simulink model "bh_2dof_NP_CONTROLLED_compare_lagr_sm"  (R2017a)
settings: Solver=ode45  StartTime=0.0  StopTime=70  FixedStep=0.001  RelTol=1e-7  EnableMultiTasking=on
values from neighbouring files (symbols this model uses):
  theta1_0 = 0    [bh_SIMPARAMS_for_2dof_NP_Control_sim.m]
  theta1_dot_0 = 0    [bh_SIMPARAMS_for_2dof_NP_Control_sim.m]
  theta4_0 = 0    [bh_SIMPARAMS_for_2dof_NP_Control_sim.m]
  theta4_dot_0 = 0    [bh_SIMPARAMS_for_2dof_NP_Control_sim.m]
undefined symbols (not defined in the file or in its folder): b1_damp, b4_damp, g, Hz, L1x, L1y, L1z, mass1, mass4, Rturn, sigbuilder_block, X, Y, Z
libraries: simulink_extras x30, sm_lib x13, nesl_utility x9, simulink x8, discretizing x2
(part 2 of 2)

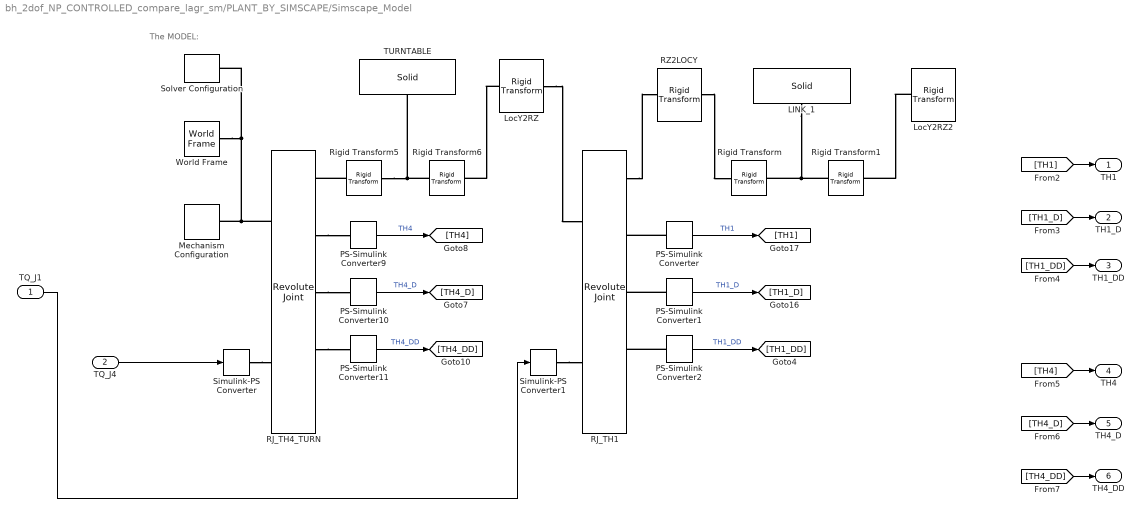
== system bh_2dof_NP_CONTROLLED_compare_lagr_sm/PLANT_BY_SIMSCAPE/Simscape_Model ==
  note: The MODEL:
  "TQ_J1 " : Inport
  TQ_J4 : Inport  Port=2
  LINK_1 : sm_lib/Body Elements/Solid  InertiaType=CalculateFromGeometry  Mass=1  MassUnits=kg  CenterOfMass=[0 0 0]  CenterOfMassUnits=m  MomentsOfInertia=[1 1 1]  MomentsOfInertiaUnits=kg*m^2  ProductsOfInertia=[0 0 0]  ProductsOfInertiaUnits=kg*m^2  DensityBased=on  Density=density  DensityUnits=kg/(m^3)  DoExposeReferenceFrame=on  SerializedFrames=<Frames/>  GraphicType=FromGeometry  MarkerShape=Sphere  MarkerSize=10  GraphicVisPropType=SimpleVisualProperties  GraphicDiffuseColor=[0.2 0.2 1.0]  GraphicSpecularColor=[0.5 0.5 0.5 1.0]  GraphicAmbientColor=[0.15 0.15 0.15 1.0]  GraphicEmissiveColor=[0.0 0.0 0.0 1.0]  GraphicShininess=75  GraphicOpacity=1.0  GeometryShape=Brick  RectangleSize=[1 1]  RectangleSizeUnits=m  BrickDimensions=[L1x, L1y, L1z ]  BrickDimensionUnits=m  CylinderRadius=1  CylinderRadiusUnits=m  CylinderLength=1  CylinderLengthUnits=m  SphereRadius=1  SphereRadiusUnits=m  EllipsoidRadii=[1 1 1]  EllipsoidRadiiUnits=m  ExtrusionCrossSection=[1 1; -1 1; -1 -1; 1 -1]  ExtrusionCrossSectionUnits=m  ExtrusionLength=1  ExtrusionLengthUnits=m  PolygonNumSides=3  PolygonOuterRadius=1  PolygonOuterRadiusUnits=m  ExtGeomFileType=STEP  ExtGeomFileUnits=m  RevolutionCrossSection=[1 1; 1 -1; 2 -1; 2 1]  RevolutionCrossSectionUnits=m  RevolutionExtent=Full  RevolutionAngle=180  RevolutionAngleUnits=deg
  LocY2RZ : sm_lib/Frames and Transforms/Rigid Transform  TranslationMethod=None  TranslationStandardOffset=Hz/2  TranslationLengthUnit=m  TranslationStandardAxis=+Z  TranslationCartesianOffset=[0 0 0]  TranslationROffset=0  TranslationROffsetUnits=m  TranslationZOffset=0  TranslationZOffsetUnits=m  TranslationThetaOffset=0  TranslationThetaOffsetUnits=deg  RotationMethod=AlignedAxes  RotationAngleUnits=deg  RotationStandardAxis=+Z  RotationAngle=0.0  RotationArbitraryAxis=[0 0 1]  FollAlignAxisA=+X  BaseAlignAxisA=+Y  FollAlignAxisB=+Y  BaseAlignAxisB=+Z  RotationSequenceAxes=FollowerAxes  RotationSequence=XYX  RotationSequenceAngles=[0 0 0]  RotationSequenceAnglesUnits=deg  RotationMatrix=[1 0 0; 0 1 0; 0 0 1]
  LocY2RZ2 : sm_lib/Frames and Transforms/Rigid Transform  TranslationMethod=None  TranslationStandardOffset=Hz/2  TranslationLengthUnit=m  TranslationStandardAxis=+Z  TranslationCartesianOffset=[0 0 0]  TranslationROffset=0  TranslationROffsetUnits=m  TranslationZOffset=0  TranslationZOffsetUnits=m  TranslationThetaOffset=0  TranslationThetaOffsetUnits=deg  RotationMethod=AlignedAxes  RotationAngleUnits=deg  RotationStandardAxis=+Z  RotationAngle=0.0  RotationArbitraryAxis=[0 0 1]  FollAlignAxisA=+X  BaseAlignAxisA=+Y  FollAlignAxisB=+Y  BaseAlignAxisB=+Z  RotationSequenceAxes=FollowerAxes  RotationSequence=XYX  RotationSequenceAngles=[0 0 0]  RotationSequenceAnglesUnits=deg  RotationMatrix=[1 0 0; 0 1 0; 0 0 1]
  Mechanism Configuration : sm_lib/Utilities/Mechanism Configuration  UniformGravity=Constant  GravityVector=[0 0 -g ]  GravityUnits=m/s^2  LinearizationDelta=1e-4
  PS-Simulink Converter : nesl_utility/PS-Simulink Converter  PhysicalDomain=network_engine_domain  SubClassName=ps_output  LeftPortType=input  RightPortType=output  PseudoPeriodic=off  Frequencies=[]  Unit=rad  AffineConversion=off
  PS-Simulink Converter1 : nesl_utility/PS-Simulink Converter  PhysicalDomain=network_engine_domain  SubClassName=ps_output  LeftPortType=input  RightPortType=output  PseudoPeriodic=off  Frequencies=[]  Unit=rad/s  AffineConversion=off
  PS-Simulink Converter10 : nesl_utility/PS-Simulink Converter  PhysicalDomain=network_engine_domain  SubClassName=ps_output  LeftPortType=input  RightPortType=output  PseudoPeriodic=off  Frequencies=[]  Unit=rad/s  AffineConversion=off
  PS-Simulink Converter11 : nesl_utility/PS-Simulink Converter  PhysicalDomain=network_engine_domain  SubClassName=ps_output  LeftPortType=input  RightPortType=output  PseudoPeriodic=off  Frequencies=[]  Unit=rad/s^2  AffineConversion=off
  PS-Simulink Converter2 : nesl_utility/PS-Simulink Converter  PhysicalDomain=network_engine_domain  SubClassName=ps_output  LeftPortType=input  RightPortType=output  PseudoPeriodic=off  Frequencies=[]  Unit=rad/s^2  AffineConversion=off
  PS-Simulink Converter9 : nesl_utility/PS-Simulink Converter  PhysicalDomain=network_engine_domain  SubClassName=ps_output  LeftPortType=input  RightPortType=output  PseudoPeriodic=off  Frequencies=[]  Unit=rad  AffineConversion=off
  RJ_TH1 : sm_lib/Joints/Revolute Joint  SenseConstraintForce=on  SenseConstraintForceX=off  SenseConstraintForceY=off  SenseConstraintForceZ=off  SenseConstraintTorque=off  SenseConstraintTorqueX=off  SenseConstraintTorqueY=off  SenseConstraintTorqueZ=off  SenseTotalForce=off  SenseTotalForceX=off  SenseTotalForceY=off  SenseTotalForceZ=off  SenseTotalTorque=off  SenseTotalTorqueX=off  SenseTotalTorqueY=off  SenseTotalTorqueZ=off  CompositeWrenchDir=BaseOnFollower  CompositeWrenchFrame=BaseFrame  EquilibriumPosition=0  EquilibriumPositionUnits=deg  SpringStiffness=0  SpringStiffnessUnits=N*m/deg  DampingCoefficient=b1_damp  DampingCoefficientUnits=N*m/(rad/s)  TorqueActuationMode=InputTorque  MotionActuationMode=ComputedMotion  SensePosition=on  SenseVelocity=on  SenseAcceleration=on  SenseTorqueForce=off  PositionTargetSpecify=on  PositionTargetPriority=Low  PositionTargetValue=theta1_0  PositionTargetValueUnits=rad  VelocityTargetSpecify=on  VelocityTargetPriority=High  VelocityTargetValue=theta1_dot_0  VelocityTargetValueUnits=rad/s
      settings: AttributesFormatString=|
      | %<DampingCoefficient>
      | %<PositionTargetValue>
      | %<VelocityTargetValue>
  RJ_TH4_TURN : sm_lib/Joints/Revolute Joint  SenseConstraintForce=on  SenseConstraintForceX=off  SenseConstraintForceY=off  SenseConstraintForceZ=off  SenseConstraintTorque=off  SenseConstraintTorqueX=off  SenseConstraintTorqueY=off  SenseConstraintTorqueZ=off  SenseTotalForce=off  SenseTotalForceX=off  SenseTotalForceY=off  SenseTotalForceZ=off  SenseTotalTorque=off  SenseTotalTorqueX=off  SenseTotalTorqueY=off  SenseTotalTorqueZ=off  CompositeWrenchDir=BaseOnFollower  CompositeWrenchFrame=BaseFrame  EquilibriumPosition=0  EquilibriumPositionUnits=deg  SpringStiffness=0  SpringStiffnessUnits=N*m/deg  DampingCoefficient=b4_damp  DampingCoefficientUnits=N*m/(rad/s)  TorqueActuationMode=InputTorque  MotionActuationMode=ComputedMotion  SensePosition=on  SenseVelocity=on  SenseAcceleration=on  SenseTorqueForce=off  PositionTargetSpecify=on  PositionTargetPriority=Low  PositionTargetValue=theta4_0  PositionTargetValueUnits=rad  VelocityTargetSpecify=on  VelocityTargetPriority=High  VelocityTargetValue=theta4_dot_0  VelocityTargetValueUnits=rad/s
      settings: AttributesFormatString=|
      | %<DampingCoefficient>
      | %<PositionTargetValue>
      | %<VelocityTargetValue>
  RZ2LOCY : sm_lib/Frames and Transforms/Rigid Transform  TranslationMethod=None  TranslationStandardOffset=Hz/2  TranslationLengthUnit=m  TranslationStandardAxis=+Z  TranslationCartesianOffset=[0 0 0]  TranslationROffset=0  TranslationROffsetUnits=m  TranslationZOffset=0  TranslationZOffsetUnits=m  TranslationThetaOffset=0  TranslationThetaOffsetUnits=deg  RotationMethod=AlignedAxes  RotationAngleUnits=deg  RotationStandardAxis=+Z  RotationAngle=0.0  RotationArbitraryAxis=[0 0 1]  FollAlignAxisA=+Y  BaseAlignAxisA=+X  FollAlignAxisB=+X  BaseAlignAxisB=+Z  RotationSequenceAxes=FollowerAxes  RotationSequence=XYX  RotationSequenceAngles=[0 0 0]  RotationSequenceAnglesUnits=deg  RotationMatrix=[1 0 0; 0 1 0; 0 0 1]
  Rigid Transform : sm_lib/Frames and Transforms/Rigid Transform  TranslationMethod=StandardAxis  TranslationStandardOffset=L1y/2  TranslationLengthUnit=m  TranslationStandardAxis=+Y  TranslationCartesianOffset=[0 0 0]  TranslationROffset=0  TranslationROffsetUnits=m  TranslationZOffset=0  TranslationZOffsetUnits=m  TranslationThetaOffset=0  TranslationThetaOffsetUnits=deg  RotationMethod=None  RotationAngleUnits=deg  RotationStandardAxis=+Z  RotationAngle=0.0  RotationArbitraryAxis=[0 0 1]  FollAlignAxisA=+X  BaseAlignAxisA=+Y  FollAlignAxisB=+Y  BaseAlignAxisB=+Z  RotationSequenceAxes=FollowerAxes  RotationSequence=XYX  RotationSequenceAngles=[0 0 0]  RotationSequenceAnglesUnits=deg  RotationMatrix=[1 0 0; 0 1 0; 0 0 1]
  Rigid Transform1 : sm_lib/Frames and Transforms/Rigid Transform  TranslationMethod=StandardAxis  TranslationStandardOffset=L1y/2  TranslationLengthUnit=m  TranslationStandardAxis=+Y  TranslationCartesianOffset=[0 0 0]  TranslationROffset=0  TranslationROffsetUnits=m  TranslationZOffset=0  TranslationZOffsetUnits=m  TranslationThetaOffset=0  TranslationThetaOffsetUnits=deg  RotationMethod=None  RotationAngleUnits=deg  RotationStandardAxis=+Z  RotationAngle=0.0  RotationArbitraryAxis=[0 0 1]  FollAlignAxisA=+X  BaseAlignAxisA=+Y  FollAlignAxisB=+Y  BaseAlignAxisB=+Z  RotationSequenceAxes=FollowerAxes  RotationSequence=XYX  RotationSequenceAngles=[0 0 0]  RotationSequenceAnglesUnits=deg  RotationMatrix=[1 0 0; 0 1 0; 0 0 1]
  Rigid Transform5 : sm_lib/Frames and Transforms/Rigid Transform  TranslationMethod=StandardAxis  TranslationStandardOffset=Hz/2  TranslationLengthUnit=m  TranslationStandardAxis=-Z  TranslationCartesianOffset=[0 0 0]  TranslationROffset=0  TranslationROffsetUnits=m  TranslationZOffset=0  TranslationZOffsetUnits=m  TranslationThetaOffset=0  TranslationThetaOffsetUnits=deg  RotationMethod=None  RotationAngleUnits=deg  RotationStandardAxis=+Z  RotationAngle=0.0  RotationArbitraryAxis=[0 0 1]  FollAlignAxisA=+X  BaseAlignAxisA=+Y  FollAlignAxisB=+Y  BaseAlignAxisB=+Z  RotationSequenceAxes=FollowerAxes  RotationSequence=XYX  RotationSequenceAngles=[0 0 0]  RotationSequenceAnglesUnits=deg  RotationMatrix=[1 0 0; 0 1 0; 0 0 1]
  Rigid Transform6 : sm_lib/Frames and Transforms/Rigid Transform  TranslationMethod=StandardAxis  TranslationStandardOffset=Hz/2  TranslationLengthUnit=m  TranslationStandardAxis=+Z  TranslationCartesianOffset=[0 0 0]  TranslationROffset=0  TranslationROffsetUnits=m  TranslationZOffset=0  TranslationZOffsetUnits=m  TranslationThetaOffset=0  TranslationThetaOffsetUnits=deg  RotationMethod=None  RotationAngleUnits=deg  RotationStandardAxis=+Z  RotationAngle=0.0  RotationArbitraryAxis=[0 0 1]  FollAlignAxisA=+X  BaseAlignAxisA=+Y  FollAlignAxisB=+Y  BaseAlignAxisB=+Z  RotationSequenceAxes=FollowerAxes  RotationSequence=XYX  RotationSequenceAngles=[0 0 0]  RotationSequenceAnglesUnits=deg  RotationMatrix=[1 0 0; 0 1 0; 0 0 1]
  Simulink-PS Converter : nesl_utility/Simulink-PS Converter  PhysicalDomain=network_engine_domain  SubClassName=ps_input  LeftPortType=input  RightPortType=output  PseudoPeriodic=off  Frequencies=[]  NoiseDistribution=none  NoiseParameters=[]  Unit=N*m  AffineConversion=off  FilteringAndDerivatives=zero  SimscapeFilterOrder=1  InputFilterTimeConstant=0.001  UdotUserProvided=1
  Simulink-PS Converter1 : nesl_utility/Simulink-PS Converter  PhysicalDomain=network_engine_domain  SubClassName=ps_input  LeftPortType=input  RightPortType=output  PseudoPeriodic=off  Frequencies=[]  NoiseDistribution=none  NoiseParameters=[]  Unit=N*m  AffineConversion=off  FilteringAndDerivatives=zero  SimscapeFilterOrder=1  InputFilterTimeConstant=0.001  UdotUserProvided=1
  Solver Configuration : nesl_utility/Solver Configuration  PhysicalDomain=network_engine_domain  SubClassName=solver  LeftPortType=input  RightPortType=generic  Accelerate=off  Tones=[]  Harmonics=[]  SimulateNoise=off  Profile=off  UseLocalSampling=off  EnableSwitchedLinearOptims=on  FrequencyDomain=off  UseCCode=off  RelTol=0.001  AbsTol=1e-06  MinStep=1e-09  ToWorkspace=off  RevertToSquareIcSolve=off  NumHomotopyIterations=100  PhasorMode=off  PhasorModeNumHarmonics=1  OverrideAbsTol=off  DoDC=off  ResidualTolerance=1e-09  UseLocalSolver=off  LocalSolverChoice=NE_TRAPEZOIDAL_ADVANCER  LocalSolverSampleTime=0.01  DoFixedCost=off  MaxNonlinIter=3  MaxModeIter=2  LinearAlgebra=Sparse  DelaysMemoryBudget=1024  AutomaticFiltering=off  FilteringTimeConstant=0.001
  TURNTABLE : sm_lib/Body Elements/Solid  InertiaType=CalculateFromGeometry  Mass=1  MassUnits=kg  CenterOfMass=[0 0 0]  CenterOfMassUnits=m  MomentsOfInertia=[1 1 1]  MomentsOfInertiaUnits=kg*m^2  ProductsOfInertia=[0 0 0]  ProductsOfInertiaUnits=kg*m^2  DensityBased=on  Density=density  DensityUnits=kg/(m^3)  DoExposeReferenceFrame=on  SerializedFrames=<Frames/>  GraphicType=FromGeometry  MarkerShape=Sphere  MarkerSize=10  GraphicVisPropType=SimpleVisualProperties  GraphicDiffuseColor=[1.0 1.0 0.2]  GraphicSpecularColor=[0.5 0.5 0.5 1.0]  GraphicAmbientColor=[0.15 0.15 0.15 1.0]  GraphicEmissiveColor=[0.0 0.0 0.0 1.0]  GraphicShininess=75  GraphicOpacity=1.0  GeometryShape=Cylinder  RectangleSize=[1 1]  RectangleSizeUnits=m  BrickDimensions=[1 1 1]  BrickDimensionUnits=m  CylinderRadius=Rturn  CylinderRadiusUnits=m  CylinderLength=Hz  CylinderLengthUnits=m  SphereRadius=1  SphereRadiusUnits=m  EllipsoidRadii=[1 1 1]  EllipsoidRadiiUnits=m  ExtrusionCrossSection=[1 1; -1 1; -1 -1; 1 -1]  ExtrusionCrossSectionUnits=m  ExtrusionLength=1  ExtrusionLengthUnits=m  PolygonNumSides=3  PolygonOuterRadius=1  PolygonOuterRadiusUnits=m  ExtGeomFileType=STEP  ExtGeomFileUnits=m  RevolutionCrossSection=[1 1; 1 -1; 2 -1; 2 1]  RevolutionCrossSectionUnits=m  RevolutionExtent=Full  RevolutionAngle=180  RevolutionAngleUnits=deg
  World Frame : sm_lib/Frames and Transforms/World Frame
  TH1 : Outport
  TH1_D : Outport  Port=2
  TH1_DD : Outport  Port=3
  TH4 : Outport  Port=4
  TH4_D : Outport  Port=5
  TH4_DD : Outport  Port=6
  wires:
  PS-Simulink Converter/1 -> [TH1]  "TH1"
  PS-Simulink Converter2/1 -> [TH1_DD]  "TH1_DD"
  PS-Simulink Converter1/1 -> [TH1_D]  "TH1_D"
  PS-Simulink Converter9/1 -> [TH4]  "TH4"
  PS-Simulink Converter11/1 -> [TH4_DD]  "TH4_DD"
  PS-Simulink Converter10/1 -> [TH4_D]  "TH4_D"
  TQ_J4/1 -> Simulink-PS Converter/1
  "TQ_J1 "/1 -> Simulink-PS Converter1/1
  [TH1] -> TH1/1
  [TH1_D] -> TH1_D/1
  [TH1_DD] -> TH1_DD/1
  [TH4_DD] -> TH4_DD/1
  [TH4_D] -> TH4_D/1
  [TH4] -> TH4/1
  connections:
  Mechanism Configuration/RConn1 -- RJ_TH4_TURN/LConn1 -- Solver Configuration/RConn1 -- World Frame/RConn1
  Rigid Transform6/LConn1 -- TURNTABLE/RConn1 -- Rigid Transform5/RConn1
  LINK_1/RConn1 -- Rigid Transform/RConn1 -- Rigid Transform1/LConn1
  Simulink-PS Converter1/RConn1 -- RJ_TH1/LConn2
  RZ2LOCY/RConn1 -- Rigid Transform/LConn1
  RJ_TH4_TURN/RConn3 -- PS-Simulink Converter10/LConn1
  PS-Simulink Converter1/LConn1 -- RJ_TH1/RConn3
  LocY2RZ/LConn1 -- Rigid Transform6/RConn1
  Rigid Transform5/LConn1 -- RJ_TH4_TURN/RConn1
  LocY2RZ/RConn1 -- RJ_TH1/LConn1
  LocY2RZ2/LConn1 -- Rigid Transform1/RConn1
  Simulink-PS Converter/RConn1 -- RJ_TH4_TURN/LConn2
  PS-Simulink Converter2/LConn1 -- RJ_TH1/RConn4
  RJ_TH1/RConn1 -- RZ2LOCY/LConn1
  RJ_TH4_TURN/RConn4 -- PS-Simulink Converter11/LConn1
  RJ_TH4_TURN/RConn2 -- PS-Simulink Converter9/LConn1
  PS-Simulink Converter/LConn1 -- RJ_TH1/RConn2

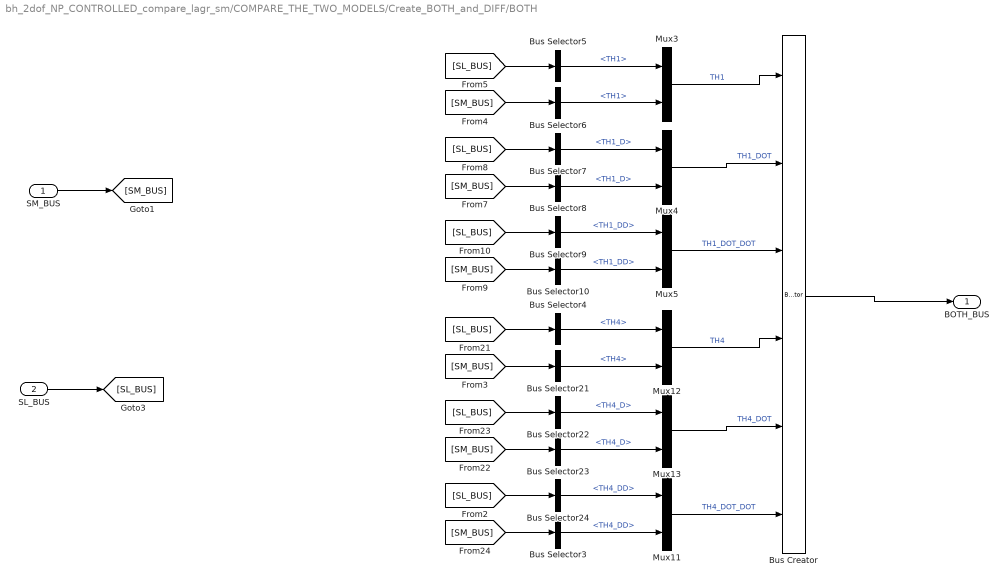
== system bh_2dof_NP_CONTROLLED_compare_lagr_sm/COMPARE_THE_TWO_MODELS/Create_BOTH_and_DIFF/BOTH ==
  SM_BUS : Inport
  SL_BUS : Inport  Port=2
  Bus Creator : BusCreator  Inputs=6
  Bus Selector10 : BusSelector  OutputSignals=TH1_DD
  Bus Selector21 : BusSelector  OutputSignals=TH4
  Bus Selector22 : BusSelector  OutputSignals=TH4_D
  Bus Selector23 : BusSelector  OutputSignals=TH4_D
  Bus Selector24 : BusSelector  OutputSignals=TH4_DD
  Bus Selector3 : BusSelector  OutputSignals=TH4_DD
  Bus Selector4 : BusSelector  OutputSignals=TH4
  Bus Selector5 : BusSelector  OutputSignals=TH1
  Bus Selector6 : BusSelector  OutputSignals=TH1
  Bus Selector7 : BusSelector  OutputSignals=TH1_D
  Bus Selector8 : BusSelector  OutputSignals=TH1_D
  Bus Selector9 : BusSelector  OutputSignals=TH1_DD
  Mux{3..5,11..13} (6 alike) : Mux  Inputs=2
  BOTH_BUS : Outport
  wires:
  SL_BUS/1 -> [SL_BUS]
  SM_BUS/1 -> [SM_BUS]
  [SM_BUS] -> Bus Selector6/1
  [SL_BUS] -> Bus Selector5/1
  [SL_BUS] -> Bus Selector7/1
  [SM_BUS] -> Bus Selector8/1
  [SL_BUS] -> Bus Selector9/1
  [SM_BUS] -> Bus Selector10/1
  Bus Selector5/1 -> Mux3/1  "<TH1>"
  Bus Selector6/1 -> Mux3/2  "<TH1>"
  Bus Selector7/1 -> Mux4/1  "<TH1_D>"
  Bus Selector8/1 -> Mux4/2  "<TH1_D>"
  Bus Selector9/1 -> Mux5/1  "<TH1_DD>"
  Bus Selector10/1 -> Mux5/2  "<TH1_DD>"
  Mux3/1 -> Bus Creator/1  "TH1"
  Mux4/1 -> Bus Creator/2  "TH1_DOT"
  Bus Creator/1 -> BOTH_BUS/1
  Mux5/1 -> Bus Creator/3  "TH1_DOT_DOT"
  [SM_BUS] -> Bus Selector21/1
  [SL_BUS] -> Bus Selector4/1
  [SL_BUS] -> Bus Selector22/1
  [SM_BUS] -> Bus Selector23/1
  [SL_BUS] -> Bus Selector24/1
  Bus Selector4/1 -> Mux12/1  "<TH4>"
  Bus Selector21/1 -> Mux12/2  "<TH4>"
  Bus Selector22/1 -> Mux13/1  "<TH4_D>"
  Bus Selector23/1 -> Mux13/2  "<TH4_D>"
  Bus Selector24/1 -> Mux11/1  "<TH4_DD>"
  Mux12/1 -> Bus Creator/4  "TH4"
  Mux13/1 -> Bus Creator/5  "TH4_DOT"
  Mux11/1 -> Bus Creator/6  "TH4_DOT_DOT"
  [SM_BUS] -> Bus Selector3/1
  Bus Selector3/1 -> Mux11/2  "<TH4_DD>"

== matlab function bh_2dof_NP_CONTROLLED_compare_lagr_sm/PLANT_BY_HAND/THE_THETA_SYS_DD ==
  data: L1X_s input; theta1_DD output; L1Y_s input; L1Z_s input; R4_s input; TH1_s input; TH1D_s input; TH4D_s input; b1_s input; b4_s input; g_s input; m1_s input; m4_s input; taum1_s input; taum4_s input; theta4_DD output
function [theta1_DD,theta4_DD] = THE_THETA_SYS_DD(L1X_s,L1Y_s,L1Z_s,R4_s,TH1_s,TH1D_s,TH4D_s,b1_s,b4_s,g_s,m1_s,m4_s,taum1_s,taum4_s)
%#codegen

%    This function was generated by the Symbolic Math Toolbox version 7.2.
%    19-Jul-2017 16:42:27

theta1_DD = (taum1_s.*1.2e1-TH1D_s.*b1_s.*1.2e1-L1Y_s.*g_s.*m1_s.*cos(TH1_s).*6.0-L1Y_s.^2.*TH4D_s.^2.*m1_s.*sin(TH1_s.*2.0).*2.0+L1Z_s.^2.*TH4D_s.^2.*m1_s.*sin(TH1_s.*2.0).*(1.0./2.0))./(L1Y_s.^2.*m1_s.*4.0+L1Z_s.^2.*m1_s);
if nargout > 1
    theta4_DD = (taum4_s.*2.4e1-TH4D_s.*b4_s.*2.4e1+L1Y_s.^2.*TH1D_s.*TH4D_s.*m1_s.*sin(TH1_s.*2.0).*8.0-L1Z_s.^2.*TH1D_s.*TH4D_s.*m1_s.*sin(TH1_s.*2.0).*2.0)./(L1X_s.^2.*m1_s.*2.0+L1Y_s.^2.*m1_s.*4.0+L1Z_s.^2.*m1_s+R4_s.^2.*m4_s.*1.2e1+L1Y_s.^2.*m1_s.*cos(TH1_s.*2.0).*4.0-L1Z_s.^2.*m1_s.*cos(TH1_s.*2.0));
end
